simulink model "Filter2simulink1"  (R2019b)
settings: Solver=VariableStepAuto  StartTime=0.0  StopTime=10.0  RelTol=1e-3
settings Model: Creator=pahul  LastModifiedBy=pahul

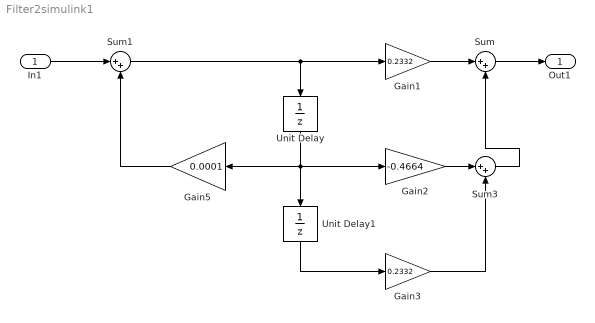
== system Filter2simulink1 ==
  In1 : Inport
  Gain1 : Gain  Gain=0.2332
  Gain2 : Gain  Gain=-0.4664
  Gain3 : Gain  Gain=0.2332
  Gain5 : Gain  Gain=0.0001
  Sum : Sum  Inputs=|++
  Sum1 : Sum  Inputs=|++
  Sum3 : Sum  Inputs=|++
  Unit Delay : UnitDelay  SampleTime=-1  HasFrameUpgradeWarning=on
  Unit Delay1 : UnitDelay  SampleTime=-1  HasFrameUpgradeWarning=on
  Out1 : Outport
  wires:
  Sum3/1 -> Sum/2
  Gain1/1 -> Sum/1
  Sum1/1 -> Gain1/1, Unit Delay/1
  Gain5/1 -> Sum1/2
  In1/1 -> Sum1/1
  Gain3/1 -> Sum3/2
  Gain2/1 -> Sum3/1
  Unit Delay1/1 -> Gain3/1
  Sum/1 -> Out1/1
  Unit Delay/1 -> Unit Delay1/1, Gain5/1, Gain2/1
